simulink subsystem "consensusPump"  (R2022b)
settings: Solver=VariableStepAuto  StartTime=0.0  StopTime=10.0  RelTol=1e-3
model mask{n_unit=0}
  mask prompts: n_unit "n_unit value"
undefined symbols (not defined in the file): c
settings Model: Creator=is123  LastModifiedBy=is123

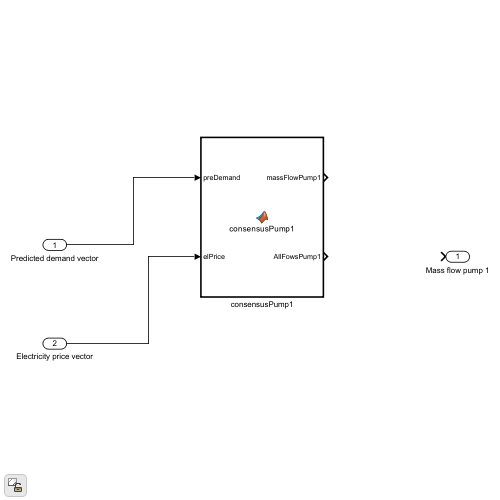
[thumbnail: Simulink's stored preview of the top-level diagram]
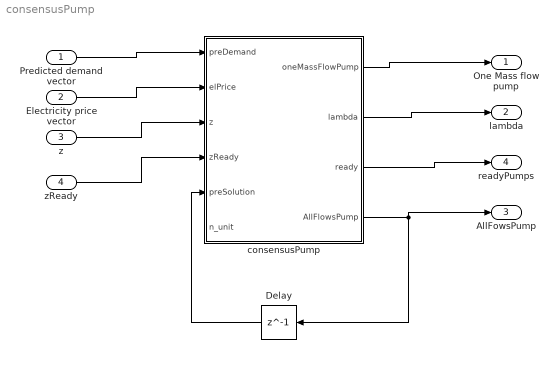
== system consensusPump ==
  Predicted demand vector : Inport
  Electricity price vector : Inport  Port=2
  z : Inport  Port=3
  zReady : Inport  Port=4
  Delay : Delay  DelayLength=1  InitialCondition=zeros(c.Nu*c.Nc,1)
  consensusPump : MATLAB Function  TreatAsAtomicUnit=on  SystemSampleTime=3600/c.AccTime
  "One Mass flow pump " : Outport
  lambda : Outport  Port=2
  "AllFowsPump " : Outport  Port=3
  readyPumps : Outport  Port=4
  wires:
  Predicted demand vector/1 -> consensusPump/1(preDemand)
  Electricity price vector/1 -> consensusPump/2(elPrice)
  consensusPump/1(oneMassFlowPump) -> "One Mass flow pump "/1
  consensusPump/4(AllFlowsPump) -> Delay/1, "AllFowsPump "/1
  z/1 -> consensusPump/3(z)
  Delay/1 -> consensusPump/5(preSolution)
  consensusPump/2(lambda) -> lambda/1
  consensusPump/3(ready) -> readyPumps/1
  zReady/1 -> consensusPump/4(zReady)

== matlab function consensusPump/consensusPump ==
  data: preDemand input; oneMassFlowPump output; lambda output; ready output; AllFlowsPump output; elPrice input; z input; zReady input; preSolution input; n_unit input
function [oneMassFlowPump,lambda,ready,AllFlowsPump] = consensusPump(preDemand, elPrice,z,zReady,preSolution,n_unit)
   %Setting up inital value of lambda
%     persistent lambda; % Declare a persistent variable
%     if isempty(lambda)
%         lambda = zeros(c.Nc*c.Nu,1);  % Set initial value
%     end
coder.extrinsic('u_consensus_fmincon')

%Getting the pump number from the mask: 

   c=scaled_standard_constants; 
   data.Je=elPrice; 
   data.d=preDemand; 
data.A_1=zeros(c.Nc,c.Nu*c.Nc);
index=1; 
for i=1:c.Nc
    data.A_1(i,index:index+c.Nu-1) = 1;
    index=index+c.Nu;
end

%Lower trangiular matrix to add consumption and flows 
data.A_2 = tril(ones(c.Nc,c.Nc));


%Making vi vectors utilized to pick out 1 of the 3 pumps values, add them up
%used to make extration limit. 
data.v1=ones(c.Nu*c.Nc,1);
data.v1(2:2:end) =0; 

data.v2=ones(c.Nu*c.Nc,1);
data.v2(1:2:end) =0;

%Making matrix which picks out 1 of the pumps for the enitre control
%horizion

data.A_31=zeros(c.Nc,c.Nu*c.Nc);
index=1; 
for i=1:c.Nc
    data.A_31(i,index) = 1;
    index=index+c.Nu;
end

data.A_32=zeros(c.Nc,c.Nu*c.Nc);
index=2; 
for i=1:c.Nc
    data.A_32(i,index) = 1;
    index=index+c.Nu;
end

  lambda = zeros(c.Nc*c.Nu,1);
  AllFlowsPump=zeros(c.Nc*c.Nu,1);
    for k=1:c.iteration
        %Telling the others that we have not yet solved the optimization
        %problem and therefore an new z value can not be determinted! 
        ready=0;
        %Updating lambda 
        if k==1 
            lambda = zeros(c.Nc*c.Nu,1);
            AllFlowsPump=[preSolution(2:end);preSolution(end,end)]; 
        else 
            lambda=lambda+c.rho*(AllFlowsPump-z); 
        end 

        %skal laves om i funktion således den ikke har brug for c
        %(forhåbenligt) 

        AllFlowsPump=u_consensus_fmincon(lambda, data, z, n_unit,AllFlowsPump);
        
        %Tells the rest that we have solved the optimization problem: 
        ready=1; 
        
        %Waiting for a update value on z 
        while zReady==0 
             
        end 
oneMassFlowPump=AllFlowsPump(n_unit,1);

    end
